simulink model "sldemo_wheelspeed_absbrake"  (R2026a)
settings: Solver=FixedStepAuto  StopTime=50  FixedStep=0.01  MaxStep=.01  AbsTol=1e-6
model workspace (MAT data in the model file):
  I = 5
  Kf = 0.8
  PBmax = 2000
  Rr = 0.4
  TB = 0.01
  v0 = 28
undefined symbols (not defined in the file or in its folder): DiscIntNeverNeededParam
Description:
  | Anti-Lock Braking System (ABS) Simulation
  | 
  | This example describes a simple model for an Anti-Lock Braking System (ABS).
  | The model sldemo_absbrake simulates the dynamic behavior of a vehicle
  | under hard braking conditions. The model represents a single wheel, which
  | may be replicated a number of times to create a model for a multi-wheel vehicle.
  | 
  | This model uses the signal logging feature in Simulink. Signals are logged to the
  | MATLAB workspace where they can be analyzed and viewed. You can view
  | the code in sldemo_absbrakeplots.m to see how this is done.
  | 
  | A detailed review of the equations used in this design can be found in
  | the white paper 'Using Simulink and Stateflow in Automotive Applications.'
settings Model: ModifiedByFormat=The MathWorks, Inc.  ExtModeTrigMode=oneshot  ExtModeArmWhenConnect=off  ExtModeAutoUpdateStatusClock=off  Creator=The MathWorks, Inc.  LastModifiedBy=The MathWorks, Inc.
settings DataIOCC: TimeSaveName=time
settings OptimizationCC: UseDivisionForNetSlopeComputation=on  InlineInvariantSignals=on  InitFltsAndDblsToZero=on  BufferReusableBoundary=off
settings DebuggingCC: SaveWithParameterizedLinksMsg=none  MultiTaskDSMMsg=warning  SigSpecEnsureSampleTimeMsg=none  IntegerOverflowMsg=none  BusObjectLabelMismatch=none  ModelReferenceSymbolNameMessage=none  SubsystemReferenceDiagnosticForUnitTest=warning  IntegerSaturationMsg=none
settings HardwareCC: ProdHWDeviceType=32-bit Generic  TargetBitPerPointer=64.0  TargetBitPerSizeT=64.0  TargetBitPerPtrDiffT=64.0  TargetLongLongMode=on  TargetIntDivRoundTo=Zero  TargetEndianess=LittleEndian  TargetWordSize=64.0  TargetHWDeviceType=MATLAB Host
settings ModelReferenceCC: ModelReferenceMinAlgLoopOccurrences=on  SupportModelReferenceSimTargetCustomCode=on
settings RTWCC: SystemTargetFile=rsim.tlc  TemplateMakefile=rsim_default_tmf  Description=Rapid Simulation Target
settings STFCustomTargetCC: SystemTargetFile=rsim.tlc  MultiwordLength=2048.0  ModelReferenceCompliant=off  MATLABClassNameForMDSCustomization=Simulink.SoftwareTarget.TargetSpecificTriggerConfigurationBase
settings RSimTargetCC: ExtModeTransport=0.0  ExtModeStaticAllocSize=1000000.0  TargetFcnLib=ansi_tfl_tmw.mat  MultiwordLength=2048.0

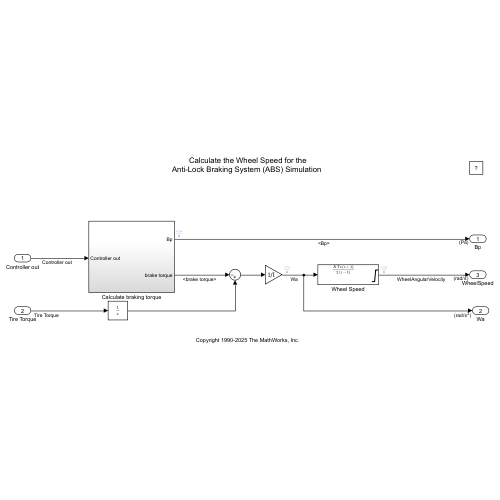
[thumbnail: Simulink's stored preview of the top-level diagram]
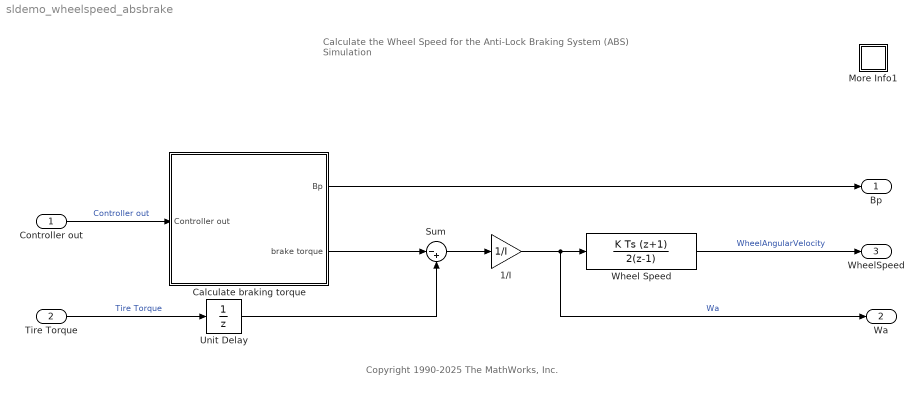
== system sldemo_wheelspeed_absbrake ==
  note: Calculate the Wheel Speed for the
      | Anti-Lock Braking System (ABS) Simulation
  note: Copyright 1990-2025 The MathWorks, Inc.
  Controller out : Inport  SampleTime=0
  Tire Torque : Inport  Port=2
  1/I : Gain  Gain=1/I  SaturateOnIntegerOverflow=on  OutDataTypeStr=Inherit: Same as input  ParamDataTypeStr=Inherit: Same as input
  Calculate braking torque : Subsystem
  More Info1 : Subsystem
      settings: OpenFcn=showExample('simulink_automotive/ModelingAnAntiLockBrakingSystemExample')
      mask Display: disp('?')
  Sum : Sum  Inputs=|-+  InputSameDT=on  SaturateOnIntegerOverflow=on  OutDataTypeStr=Inherit: Same as first input
  Unit Delay : UnitDelay  SampleTime=-1
  Wheel Speed : DiscreteIntegrator  IntegratorMethod=Integration: Trapezoidal  InitialCondition=v0/Rr  SampleTime=-1  LimitOutput=on  UpperSaturationLimit=1000  LowerSaturationLimit=0  ICPrevOutput=DiscIntNeverNeededParam  ICPrevScaledInput=DiscIntNeverNeededParam
  Bp : Outport  Unit=Pa
  Wa : Outport  Port=2  Unit=rad/s^2
  WheelSpeed : Outport  Port=3  Unit=rad/s  VectorParamsAs1DForOutWhenUnconnected=off
  wires:
  1/I/1 -> Wheel Speed/1, Wa/1  "Wa"
  Sum/1 -> 1/I/1
  Tire Torque/1 -> Unit Delay/1  "Tire Torque"
  Controller out/1 -> Calculate braking torque/1(Controller out)  "Controller out"
  Calculate braking torque/2(brake torque) -> Sum/1
  Calculate braking torque/1(Bp) -> Bp/1
  Unit Delay/1 -> Sum/2
  Wheel Speed/1 -> WheelSpeed/1  "WheelAngularVelocity"

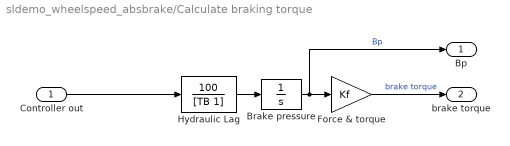
== system sldemo_wheelspeed_absbrake/Calculate braking torque ==
  Controller out : Inport
  Brake pressure : Integrator  LimitOutput=on  UpperSaturationLimit=PBmax  LowerSaturationLimit=0
  Force & torque : Gain  Gain=Kf  SaturateOnIntegerOverflow=on  OutDataTypeStr=Inherit: Same as input  ParamDataTypeStr=Inherit: Same as input
  "Hydraulic Lag " : TransferFcn  Numerator=[100]  Denominator=[TB 1]
  Bp : Outport
  brake torque : Outport  Port=2
  wires:
  "Hydraulic Lag "/1 -> Brake pressure/1
  Brake pressure/1 -> Bp/1, Force & torque/1  "Bp"
  Force & torque/1 -> brake torque/1  "brake torque"
  Controller out/1 -> "Hydraulic Lag "/1

== system sldemo_wheelspeed_absbrake/More Info1 ==
